simulink model "simSpd"  (R2016b)
settings: Solver=ode45  StartTime=0.0  StopTime=40  RelTol=1e-3  EnableMultiTasking=on
values from neighbouring files (symbols this model uses):
  Arm = 0.5    [system_constants_and_controller_design.m]
  Fmax = 16    [system_constants_and_controller_design.m]
  K0 = C0.K    [system_constants_and_controller_design.m]
  Kd = 25    [system_constants_and_controller_design.m]
  KVmax = CVmax.K    [system_constants_and_controller_design.m]
  M = 0.91375475796    [system_constants_and_controller_design.m]
  motorDeadZone = 0.1    [system_constants_and_controller_design.m]
  sensorPeriod = 1/100    (= 0.01)    [system_constants_and_controller_design.m]
  Vmax = sqrt(Tmax/Kd)    [system_constants_and_controller_design.m]
libraries: simulink x2, cstblocks x1
settings Model: Creator=Cassandra  LastModifiedBy=Cassandra
settings DataIOCC: LimitDataPoints=on  SaveFormat=Array
settings OptimizationCC: LifeSpan=inf
settings DebuggingCC: MaxConsecutiveZCsMsg=none  SFUnexpectedBacktrackingDiag=warning  SFNoUnconditionalDefaultTransitionDiag=warning  SFExecutionAtInitializationDiag=none
settings HardwareCC: ProdBitPerPointer=32  ProdBitPerSizeT=32  ProdBitPerPtrDiffT=32  ProdLargestAtomicFloat=None  ProdIntDivRoundTo=Undefined  ProdEndianess=Unspecified  ProdWordSize=32  ProdHWDeviceType=32-bit Generic
settings ModelReferenceCC: PropagateSignalLabelsOutOfModel=off
settings GRTTargetCC: TargetLangStandard=C89/C90 (ANSI)  GeneratePreprocessorConditionals=Disable all
settings ConfigComp: CovMetricSettings=dw  CovHtmlReporting=on  CovSaveCumulativeToWorkspaceVar=on  CovSaveSingleToWorkspaceVar=on  CovExternalEMLEnable=off

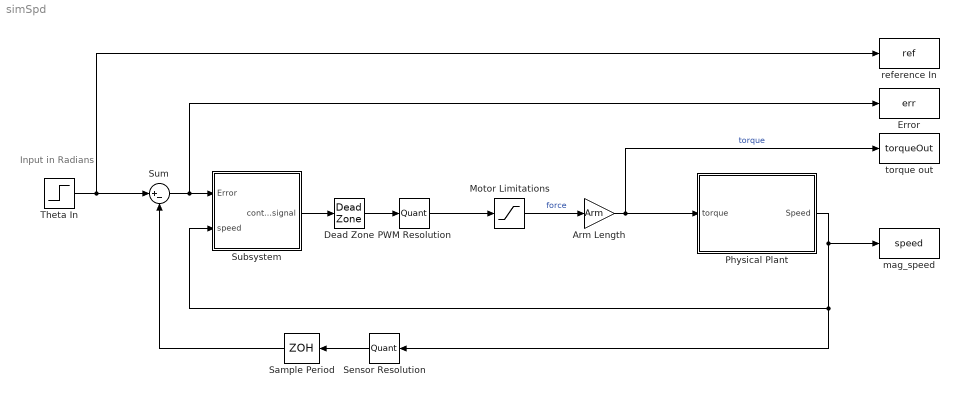
== system simSpd ==
  note: Input in Radians
  Arm Length : Gain  Gain=Arm
  Dead Zone : DeadZone  LowerValue=-motorDeadZone  UpperValue=motorDeadZone  SaturateOnIntegerOverflow=on
  Error : ToWorkspace  VariableName=err  SaveFormat=Timeseries  SampleTime=-1
  Motor Limitations : Saturate  UpperLimit=Fmax  LowerLimit=-Fmax
  PWM Resolution : Quantizer  QuantizationInterval=motorResolution
  Physical Plant : Subsystem
  Sample Period : ZeroOrderHold  SampleTime=sensorPeriod
  Sensor Resolution : Quantizer  QuantizationInterval=sensorResolution
  Subsystem : Subsystem
  Sum : Sum  Inputs=|+-
  Theta In : Step  After=pi/2  SampleTime=0
  mag_speed : ToWorkspace  VariableName=speed  SaveFormat=Timeseries  SampleTime=-1
  reference In : ToWorkspace  VariableName=ref  SaveFormat=Timeseries  SampleTime=-1
  torque out : ToWorkspace  VariableName=torqueOut  SaveFormat=Timeseries  SampleTime=-1
  wires:
  Theta In/1 -> reference In/1, Sum/1
  PWM Resolution/1 -> Motor Limitations/1
  Sensor Resolution/1 -> Sample Period/1
  Sum/1 -> Subsystem/1(Error), Error/1
  Arm Length/1 -> Physical Plant/1(torque), torque out/1  "torque"
  Sample Period/1 -> Sum/2
  Motor Limitations/1 -> Arm Length/1  "force"
  Dead Zone/1 -> PWM Resolution/1
  Subsystem/1(control signal) -> Dead Zone/1
  Physical Plant/1(Speed) -> Sensor Resolution/1, Subsystem/2(speed), mag_speed/1

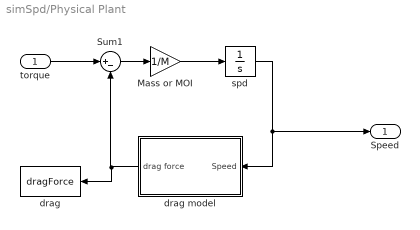
== system simSpd/Physical Plant ==
  torque : Inport
  Mass or MOI : Gain  Gain=1/M
  Sum1 : Sum  Inputs=|+-
  drag : ToWorkspace  VariableName=dragForce  SaveFormat=Timeseries  SampleTime=-1
  drag model : Subsystem
  spd : Integrator
  Speed : Outport
  wires:
  spd/1 -> drag model/1(Speed), Speed/1
  Mass or MOI/1 -> spd/1
  Sum1/1 -> Mass or MOI/1
  drag model/1(drag force) -> Sum1/2, drag/1
  torque/1 -> Sum1/1

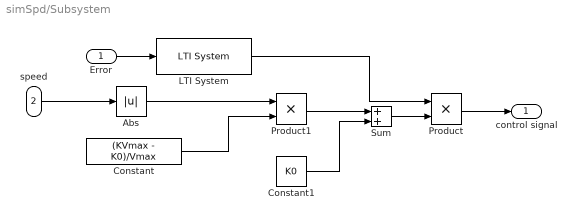
== system simSpd/Subsystem ==
  Error : Inport
  speed : Inport  Port=2
  Abs : Abs
  Constant : Constant  Value=(KVmax - K0)/Vmax
  Constant1 : Constant  Value=K0
  LTI System : cstblocks/LTI System  sys=comp  IC=[]
  Product : Product
  Product1 : Product
  Sum : Sum
  control signal : Outport
  wires:
  speed/1 -> Abs/1
  Abs/1 -> Product1/1
  Product/1 -> control signal/1
  Sum/1 -> Product/2
  Product1/1 -> Sum/1
  LTI System/1 -> Product/1
  Error/1 -> LTI System/1
  Constant1/1 -> Sum/2
  Constant/1 -> Product1/2

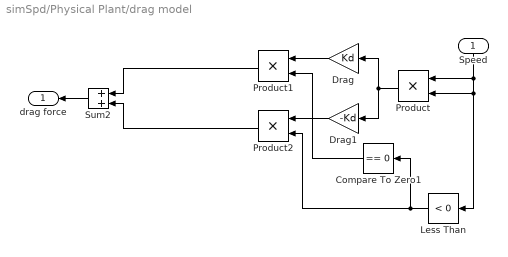
== system simSpd/Physical Plant/drag model ==
  Speed : Inport
  Compare To Zero1 : simulink/Logic and Bit Operations/Compare To Zero  relop===  OutDataTypeStr=boolean
  Drag : Gain  Gain=Kd
  Drag1 : Gain  Gain=-Kd
  Less Than : simulink/Logic and Bit Operations/Compare To Zero  relop=<  OutDataTypeStr=boolean
  Product : Product
  Product1 : Product
  Product2 : Product
  Sum2 : Sum  Inputs=+|+
  drag force : Outport
  wires:
  Speed/1 -> Product/1, Less Than/1, Product/2
  Drag1/1 -> Product2/1
  Compare To Zero1/1 -> Product1/2
  Product1/1 -> Sum2/1
  Drag/1 -> Product1/1
  Sum2/1 -> drag force/1
  Product/1 -> Drag1/1, Drag/1
  Product2/1 -> Sum2/2
  Less Than/1 -> Product2/2, Compare To Zero1/1
